simulink model "PC_MSFS_STATION"  (R2021b)
settings: Solver=FixedStepAuto  StartTime=0.0  StopTime=2000  FixedStep=0.03  RelTol=1e-3
undefined symbols (not defined in the file): CONTROL, DiscIntNeverNeededParam, f, MODEL, MODEL_INI
libraries: instrumentlib x43, SimConnectToolbox x6, simulink x4
(part 3 of 3)

== matlab function PC_MSFS_STATION/CONTROL/MEDEVAC/CONTROL UPDATE ==
  data: CONTROL_IN input; CONTROL output Bus: CONTROL_Bus; STATE input; ALTITUDE_IN input
function CONTROL = CONTROL_UPDATE(CONTROL_IN, STATE, ALTITUDE_IN)
% COPY CONTROL BUS
CONTROL = CONTROL_IN;
CONTROL.PARAM.SIM_TIME = CONTROL.PARAM.SIM_TIME + CONTROL.PARAM.SAMPLING_TIME;
curr_sim_time = CONTROL.PARAM.SIM_TIME;
deltat = CONTROL.PARAM.SAMPLING_TIME;
flight_status = CONTROL.PARAM.FLIGHT_STATUS;
timer = CONTROL.PARAM.TIMER;
sim_control_mode = CONTROL.PARAM.SIM_CONTROL_MODE;
%--------------------------------------------------------------------------
% CONTROL PARAMETERS
%--------------------------------------------------------------------------
% Nominal Control Parameters
kyd = CONTROL.PARAM.NAV_D_1;

% Navigation Variables
%altitude = ALTITUDE_IN;
altitude_control = CONTROL.PARAM.ALTITUDE_REF;
%rho = altitude + 20.902e6;

% Extra Parameters
tau_max = CONTROL.PARAM.TAU_MAX;
take_off_signal = CONTROL.PARAM.TAKE_OFF;
land_signal = CONTROL.PARAM.LANDING;
%--------------------------------------------------------------------------
% CONTROL TARGETS
%--------------------------------------------------------------------------
simu_end = CONTROL.TARGET.SIMU_END;
target_latitude = CONTROL.TARGET.LATITUDE*pi/180;
target_longitude = CONTROL.TARGET.LONGITUDE*pi/180;
snom = CONTROL.TARGET.VELOCITY;
dist_obstacle = CONTROL.PARAM.DIST_OBSTACLE;
CBF_const = CONTROL.PARAM.CBF_CONST;
obst_threatclass = CONTROL.TARGET.OBSTACLE_THREATCLASS;
waypoint_verified = CONTROL.TARGET.WAYPOINT_VERIFIED;
human_att_mode = CONTROL.TARGET.HUMAN_ATT_MODE;
%--------------------------------------------------------------------------
% CONTROL CBFS
%--------------------------------------------------------------------------
h = CONTROL.PARAM.CBF_H;
hdot = CONTROL.PARAM.CBF_HDOT;
psi = CONTROL.PARAM.CBF_PSI;
A1_qp = CONTROL.PARAM.CBF_A1QP;
A2_qp = CONTROL.PARAM.CBF_A2QP;
b1_qp = CONTROL.PARAM.CBF_B1QP;


ua_system = CONTROL.OUTPUT.UA;
ualpha_system = CONTROL.OUTPUT.UALPHA;
%--------------------------------------------------------------------------
% SYSTEM CURRENT STATE
%--------------------------------------------------------------------------
% Update Current State
y1 = STATE(1);
y2 = STATE(2);
vy1 = STATE(3);
vy2 = STATE(4);

timer = timer + deltat;

% FLIGHT STATUS 0 = INITIALIZATION
if flight_status == 0
    altitude = ALTITUDE_IN;
    rho = altitude + 20.902e6;
    % VIRTUAL NOMINAL CONTROLLER (tau1, tau2)
    tau1_nom_PD = - kyd*(vy1 - 0);
    tau2_nom_PD = - kyd*(vy2 - 0);
    tau1_applied = tau1_nom_PD;
    tau2_applied = tau2_nom_PD;
    
    if abs(tau1_applied) >= tau_max
        tau1_applied = sign(tau1_applied)*tau_max;
    else
        tau1_applied = tau1_applied;
    end
    
    if abs(tau2_applied) >= tau_max
        tau2_applied = sign(tau2_applied)*tau_max;
    else
        tau2_applied = tau2_applied;
    end
    if take_off_signal == 1
        flight_status = 1;
        timer = 0;
    end

%     if curr_sim_time >= 5
%         flight_status = 1;
%         timer = 0;
%     end 

elseif flight_status == 1
    altitude = altitude_control;
    rho = altitude + 20.902e6;
    tau1_nom_PD = - kyd*(vy1 - 0);
    tau2_nom_PD = - kyd*(vy2 - 0);
    tau1_applied = tau1_nom_PD;
    tau2_applied = tau2_nom_PD;
    
    if abs(tau1_applied) >= tau_max
        tau1_applied = sign(tau1_applied)*tau_max;
    else
        tau1_applied = tau1_applied;
    end
    
    if abs(tau2_applied) >= tau_max
        tau2_applied = sign(tau2_applied)*tau_max;
    else
        tau2_applied = tau2_applied;
    end
    if curr_sim_time >= 8
        flight_status = 2;
        timer = 0;
    end

elseif flight_status == 2
    % ON FLIGHT
    %--------------------------------------------------------------------------
    % DERIVATIVE (D) CONTROL
    %--------------------------------------------------------------------------
    altitude = altitude_control;
    rho = altitude + 20.902e6;

    wp1 = rho*cos(target_latitude)*cos(target_longitude);
    wp2 = rho*cos(target_latitude)*sin(target_longitude);
    
    % NOMINAL CONTROLLER
    % System Quadrant
    pos1_PD = wp1 - y1;
    pos2_PD = wp2 - y2;

    theta_PD = atan2(pos2_PD,pos1_PD);

%     if pos1_PD >=0
%         % First or fourth quadrant
%         if pos2_PD >=0
%             %First quadrant
%             theta_PD = atan(abs(pos2_PD)/abs(pos1_PD));
%         else
%             % Fourth quadrant
%             %                 theta_PD = 2*pi - atan(abs(pos2_PD)/abs(pos1_PD));
%             theta_PD = - atan(abs(pos2_PD)/abs(pos1_PD));
%         end
%     else
%         % Second or third quadrant
%         if pos2_PD >=0
%             % Second quadrant
%             theta_PD = pi - atan(abs(pos2_PD)/abs(pos1_PD));
%         else
%             % Third quadrant
%             theta_PD = pi + atan(abs(pos2_PD)/abs(pos1_PD));
%         end
%     end

    % New target velocity
    vs1_PD = snom*cos(theta_PD);
    vs2_PD = snom*sin(theta_PD);

    % VIRTUAL NOMINAL CONTROLLER (tau1, tau2)
    tau1_nom_PD = - kyd*(vy1 - vs1_PD);
    tau2_nom_PD = - kyd*(vy2 - vs2_PD);

    if sim_control_mode == 0
        %------------------------------------------------------------------
        % TRACKING ONLY
        %------------------------------------------------------------------
        tau1_applied = tau1_nom_PD;
        tau2_applied = tau2_nom_PD;
    else
        %------------------------------------------------------------------
        % CBF - SAFETY FILTERS: Avoid "unverified region" of target wp
        %------------------------------------------------------------------
        if (waypoint_verified == 0) % Waypoint not verified
            dist_obs_scaled = obst_threatclass*dist_obstacle;
            if (human_att_mode == 1) % Att CBFs
                alpha_val = STATE(8);
                CBF_const_att = CBF_const*alpha_val;
                CONTROL.PARAM.CBF_CONST_ATT = CBF_const_att;
            else % Standard CBF
                CBF_const_att = CBF_const;
            end
            h = (y1 - wp1)^2 + (y2 - wp2)^2 - dist_obs_scaled^2;
            hdot = 2*(y1 - wp1)*vy1 + 2*(y2 - wp2)*vy2;
            psi = hdot + CBF_const_att*h;
            A1_qp = 2*(y1 - wp1);
            A2_qp = 2*(y2 -wp2);
            b1_qp = 2*(vy1^2 + vy2^2) + CBF_const_att*hdot + CBF_const_att*psi;
            
        else % Waypoint verified
            h = 0;
            hdot = 0;
            psi = 0;
            A1_qp = 0;
            A2_qp = 0;
            b1_qp = 0;
            % REDUCE NOMINAL SPEED TO 20% FOR LANDING APPROACH AFTER
            % REMOVING CBF!!!!!!
            % New target velocity
            vs1_PD = snom*cos(theta_PD)*0.2;
            vs2_PD = snom*sin(theta_PD)*0.2;
            tau1_nom_PD = - kyd*(vy1 - vs1_PD);
            tau2_nom_PD = - kyd*(vy2 - vs2_PD);
        end

        A_qp = -[A1_qp, A2_qp];
        b_qp = [b1_qp];
        H_qp = 2*[1, 0; 0, 1];
        f_qp = -2*[tau1_nom_PD; tau2_nom_PD];
        x0_qp = [tau1_nom_PD; tau2_nom_PD];
        option_qp = optimoptions('quadprog','Algorithm','active-set','Display','None');
        [tau_applied, fval_qp, exitval_qp] = quadprog(H_qp, double(f_qp), A_qp, b_qp,[],[],[],[],x0_qp,option_qp);
        tau1_applied = tau_applied(1);
        tau2_applied = tau_applied(2);

        CONTROL.PARAM.CBF_H = h;
        CONTROL.PARAM.CBF_PSI = psi;
    end

    % UPDATE FLIGHT STATUS IF LANDING SIGNAL RECEIVED
    if land_signal == 1
        flight_status = 3;
    end

    % SATURATE CONTROL INPUT FOR SMOOTH TURNING
    s_system = STATE(5);
    theta_system = STATE(6);
    omega_system = STATE(7);
    p_system = CONTROL.PARAM.DIST_P;
    update_taus = 0;
    ua_system = tau1_applied*cos(theta_system) + tau2_applied*sin(theta_system) + p_system*omega_system^2;
    ualpha_system = -tau1_applied*sin(theta_system)/p_system + tau2_applied*cos(theta_system)/p_system - omega_system*s_system/p_system;
    
%     if (abs(ualpha_system) > 2000)
%         ualpha_system = 2000*sign(ualpha_system);
%     end
%     if (abs(ua_system) > 2000)
%         ua_system = 2000*sign(ua_system);
%         update_taus = 1;
%     end
%     if (update_taus == 1)
%         tau1_applied = ua_system*cos(theta_system) - ualpha_system*p_system*sin(theta_system) - s_system*omega_system*sin(theta_system) - p_system*omega_system^2*cos(theta_system);
%         tau2_applied = ua_system*sin(theta_system) + ualpha_system*p_system*cos(theta_system) + s_system*omega_system*cos(theta_system) - p_system*omega_system^2*sin(theta_system);
%     end
    
    if abs(tau1_applied) >= tau_max
        tau1_applied = sign(tau1_applied)*tau_max;
    else
        tau1_applied = tau1_applied;
    end

    if abs(tau2_applied) >= tau_max
        tau2_applied = sign(tau2_applied)*tau_max;
    else
        tau2_applied = tau2_applied;
    end
    
else
    %%% FLIGHT STATUS = 3 - LANDING SIGNAL RECEIVED (HOVER CONTROL)
    altitude = altitude_control;
    rho = altitude + 20.902e6;
    tau1_nom_PD = - 0*kyd*(vy1 - 0);
    tau2_nom_PD = - 0*kyd*(vy2 - 0);
    tau1_applied = tau1_nom_PD;
    tau2_applied = tau2_nom_PD;
    
    if abs(tau1_applied) >= tau_max
        tau1_applied = sign(tau1_applied)*tau_max;
    else
        tau1_applied = tau1_applied;
    end
    
    if abs(tau2_applied) >= tau_max
        tau2_applied = sign(tau2_applied)*tau_max;
    else
        tau2_applied = tau2_applied;
    end

end


%%%%%%%%%%%%%%%%%%%%%%%%%%%%%%%%%%%%%%%%%%%%%%%%%%%%%%%%%%%%%%%%%%%%%%%%%%%
% OUTPUT BUS
%%%%%%%%%%%%%%%%%%%%%%%%%%%%%%%%%%%%%%%%%%%%%%%%%%%%%%%%%%%%%%%%%%%%%%%%%%%
CONTROL.TARGET.SIMU_END = simu_end;
CONTROL.OUTPUT.TAU1 = tau1_applied;
CONTROL.OUTPUT.TAU2 = tau2_applied;

CONTROL.OUTPUT.TAU1_NOM = tau1_nom_PD;
CONTROL.OUTPUT.TAU2_NOM = tau2_nom_PD;

CONTROL.PARAM.FLIGHT_STATUS = flight_status;
CONTROL.PARAM.ALTITUDE = altitude;
CONTROL.PARAM.RHO = rho;
CONTROL.PARAM.TIMER = timer;

CONTROL.OUTPUT.UA = ua_system;
CONTROL.OUTPUT.UALPHA = ualpha_system;

return
